simulink model "Modulador_torque_compensado"  (R2020a)
settings: Solver=VariableStepAuto  StartTime=0.0  StopTime=10.0  RelTol=1e-3
undefined symbols (not defined in the file): bm, bm_virtual, g, K_motor, K_motor_virtual, L, m_total, m_total_virtual, R, R_control
settings Model: Creator=Adriana  LastModifiedBy=Adriana

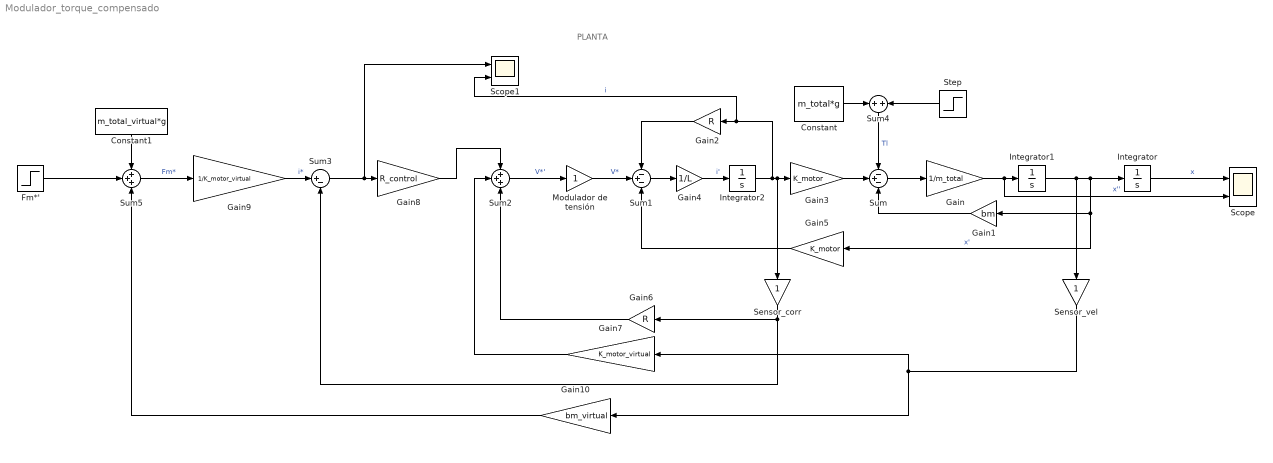
== system Modulador_torque_compensado ==
  note: PLANTA
  " Sensor_vel" : Gain
  Constant : Constant  Value=m_total*g
  Constant1 : Constant  Value=m_total_virtual*g
  Fm*' : Step  SampleTime=0
  Gain : Gain  Gain=1/m_total
  Gain1 : Gain  Gain=bm
  Gain10 : Gain  Gain=bm_virtual
  Gain2 : Gain  Gain=R
  Gain3 : Gain  Gain=K_motor
  Gain4 : Gain  Gain=1/L
  Gain5 : Gain  Gain=K_motor
  Gain6 : Gain  Gain=R
  Gain7 : Gain  Gain=K_motor_virtual
  Gain8 : Gain  Gain=R_control
  Gain9 : Gain  Gain=1/K_motor_virtual
  Integrator : Integrator
  Integrator1 : Integrator
  Integrator2 : Integrator
  Modulador de tensión : Gain
  Scope : Scope  NumInputPorts=2
  Scope1 : Scope  NumInputPorts=2
  Sensor_corr : Gain
  Step : Step  Time=3  After=0  SampleTime=0
  Sum : Sum  Inputs=-+-
  Sum1 : Sum  Inputs=-+-
  Sum2 : Sum  Inputs=+++
  Sum3 : Sum  Inputs=|+-
  Sum4 : Sum
  Sum5 : Sum  Inputs=+++
  wires:
  Integrator1/1 -> " Sensor_vel"/1, Gain5/1, Gain1/1, Integrator/1  "x'"
  Integrator/1 -> Scope/1  "x"
  Gain/1 -> Scope/2, Integrator1/1  "x''"
  Sum/1 -> Gain/1
  Gain1/1 -> Sum/3
  Sum4/1 -> Sum/1  "Tl"
  Gain3/1 -> Sum/2
  Integrator2/1 -> Scope1/2, Gain2/1, Gain3/1, Sensor_corr/1  "i"
  Sum1/1 -> Gain4/1
  Gain4/1 -> Integrator2/1  "i'"
  Gain2/1 -> Sum1/1
  Gain5/1 -> Sum1/3
  Modulador de tensión/1 -> Sum1/2  "V*"
  Sum2/1 -> Modulador de tensión/1  "V*'"
  " Sensor_vel"/1 -> Gain10/1, Gain7/1
  Sensor_corr/1 -> Sum3/2, Gain6/1
  Gain6/1 -> Sum2/3
  Gain7/1 -> Sum2/2
  Gain8/1 -> Sum2/1
  Sum3/1 -> Scope1/1, Gain8/1
  Gain9/1 -> Sum3/1  "i*"
  Step/1 -> Sum4/2
  Constant/1 -> Sum4/1
  Sum5/1 -> Gain9/1  "Fm*"
  Fm*'/1 -> Sum5/2
  Gain10/1 -> Sum5/3
  Constant1/1 -> Sum5/1
